simulink model "Testing_User_defined_Function"  (R2019b)
settings: Solver=VariableStepAuto  StartTime=0.0  StopTime=10  FixedStep=0.0001  RelTol=1e-3
values from neighbouring files (symbols this model uses):
  B = (NL_current*Km)/NL_speed    (= 7.06678023853e-07)    [DCX19_Motor_Calculations.m]
  J = 2.72*10^-7    (= 2.72e-07)    [DCX19_Motor_Calculations.m]
  Kb = 1/(268*(2*pi/60))    (= 0.0356317036773)    [DCX19_Motor_Calculations.m]
  Kd = (K - Kp)/filter_pole    [DCX19_Motor_Calculations.m]
  Ki = ((z1*z2)*K)/filter_pole    [DCX19_Motor_Calculations.m]
  Km = 35.6*10^-3    (= 0.0356)    [DCX19_Motor_Calculations.m]
  Kp = (K*(z1 + z2) - Ki)/filter_pole    [DCX19_Motor_Calculations.m]
  L = 1.320*10^-3    (= 0.00132)    [DCX19_Motor_Calculations.m]
  res = (2*pi)/CPR    (= 0.0490873852123)    [DCX19_Motor_Calculations.m]
undefined symbols (not defined in the file or in its folder): R
libraries: cstblocks x2, simulink x1
settings Model: Creator=harsh  LastModifiedBy=harsh

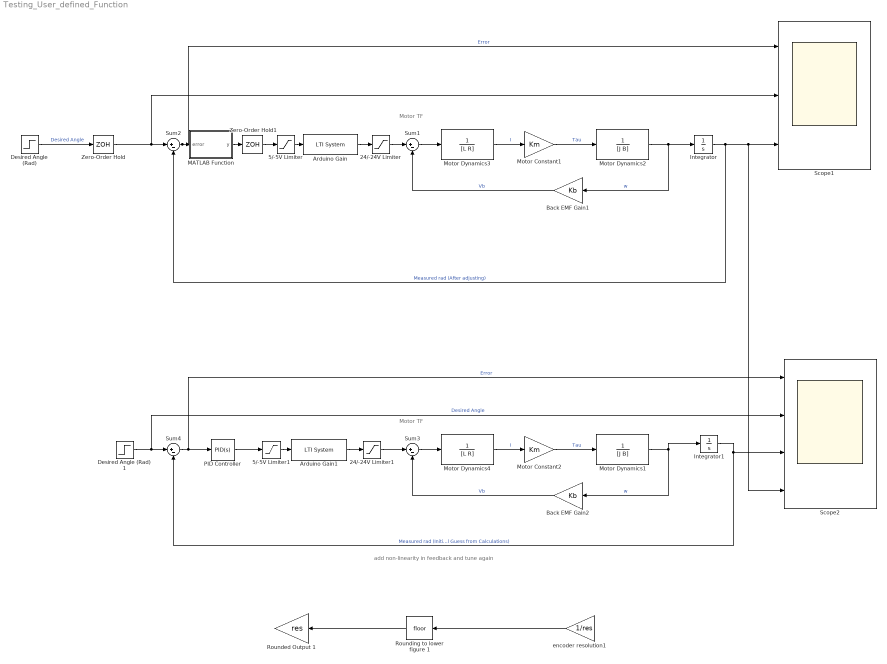
== system Testing_User_defined_Function ==
  note: add non-linearity in feedback and tune again
  note: Motor TF
  note: Motor TF
  24/-24V Limiter : Saturate  UpperLimit=5  LowerLimit=-5
  24/-24V Limiter1 : Saturate  UpperLimit=5  LowerLimit=-5
  5/-5V Limiter : Saturate  UpperLimit=5  LowerLimit=-5
  5/-5V Limiter1 : Saturate  UpperLimit=5  LowerLimit=-5
  Arduino Gain : cstblocks/LTI System  sys=OPAMP  IC=[]
  Arduino Gain1 : cstblocks/LTI System  sys=OPAMP  IC=[]
  Back EMF Gain1 : Gain  Gain=Kb
  Back EMF Gain2 : Gain  Gain=Kb
  "Desired Angle (Rad) " : Step  After=1.5707  SampleTime=0
  Desired Angle (Rad) 1 : Step  After=1.5707  SampleTime=0
  Integrator : Integrator
  Integrator1 : Integrator
  MATLAB Function : MATLAB Function  TreatAsAtomicUnit=on
  Motor Constant1 : Gain  Gain=Km
  Motor Constant2 : Gain  Gain=Km
  Motor Dynamics1 : TransferFcn  Denominator=[J B]
  Motor Dynamics2 : TransferFcn  Denominator=[J B]
  Motor Dynamics3 : TransferFcn  Denominator=[L R]
  Motor Dynamics4 : TransferFcn  Denominator=[L R]
  PID Controller : simulink/Continuous/PID Controller  Controller=PID  Form=Parallel  TimeDomain=Continuous-time  SampleTime=-1  IntegratorMethod=Forward Euler  FilterMethod=Forward Euler  ControllerParametersSource=internal  P=Kp  I=Ki  D=Kd  UseFilter=on  N=5000  TunerSelectOption=Transfer Function Based (PID Tuner App)  InitialConditionSource=internal  InitialConditionForIntegrator=0  InitialConditionForFilter=0  DifferentiatorICPrevScaledInput=0  ExternalReset=none  TrackingMode=off  Kt=1  LimitOutput=off  UpperSaturationLimit=inf  LowerSaturationLimit=-inf  LinearizeAsGain=on  AntiWindupMode=none  Kb=1  POutMin=[]  POutMax=[]  IOutMin=[]  IOutMax=[]  DOutMin=[]  DOutMax=[]  NOutMin=[]  NOutMax=[]  SumOutMin=[]  SumOutMax=[]  SaturationOutMin=[]  SaturationOutMax=[]  PParamMin=[]  PParamMax=[]  IParamMin=[]  IParamMax=[]  DParamMin=[]  DParamMax=[]  NParamMin=[]  NParamMax=[]  KbParamMin=[]  KbParamMax=[]  KtParamMin=[]  KtParamMax=[]  KbOutMin=[]  KbOutMax=[]  KtOutMin=[]  KtOutMax=[]  IntegratorOutMin=[]  IntegratorOutMax=[]  FilterOutMin=[]  FilterOutMax=[]  SumI1OutMin=[]  SumI1OutMax=[]  SumI2OutMin=[]  SumI2OutMax=[]  SumI3OutMin=[]  SumI3OutMax=[]  SumI4OutMin=[]  SumI4OutMax=[]  SumDOutMin=[]  SumDOutMax=[]  DifferentiatorOutMin=[]  DifferentiatorOutMax=[]  FilterDiffOutCoefMin=[]  FilterDiffOutCoefMax=[]  ReciprocalOutMin=[]  ReciprocalOutMax=[]  SumDenOutMin=[]  SumDenOutMax=[]  SumNumOutMin=[]  SumNumOutMax=[]  DivideOutMin=[]  DivideOutMax=[]  IntegratorContinuousStateAttributes=''  IntegratorStateMustResolveToSignalObject=off  IntegratorRTWStateStorageClass=Auto  FilterContinuousStateAttributes=''  FilterStateMustResolveToSignalObject=off  FilterRTWStateStorageClass=Auto  ParallelPVariant=InternalParameters  IdealPVariant=Disabled  IVariant=InternalParameters  DVariant=InternalParameters  IntegratorVariant=Continuous  SatVariant=Disabled  AWVariant=Passthrough  PCopyVariant=Disabled  TRVariant=Disabled  FdbkBlocksVariant=Forward  IdealPFdbkVariant=Disabled  SatFdbkVariant=Disabled  DerivativeFilterVariant=ContFilter  NVariant=InternalParameters  NCopyVariant=Disabled  FilterICVariant=InternalICsFilter  IntegratorICVariant=InternalICs  ExternalResetVariant=Disabled  TRSumVariant=Passthrough  SumFdbkVariant=Disabled  SumVariant=Sum_PID
  Rounded Output 1 : Gain  Gain=res
  Rounding to lower figure 1 : Rounding
  Scope1 : Scope  NumInputPorts=3
  Scope2 : Scope  NumInputPorts=4
  Sum{1..4} (4 alike) : Sum  Inputs=|+-
  Zero-Order Hold : ZeroOrderHold  SampleTime=0.0001
  Zero-Order Hold1 : ZeroOrderHold  SampleTime=0.0001
  encoder resolution1 : Gain  Gain=1/res
  wires:
  5/-5V Limiter/1 -> Arduino Gain/1
  Sum1/1 -> Motor Dynamics3/1
  Arduino Gain/1 -> 24/-24V Limiter/1
  Back EMF Gain1/1 -> Sum1/2  "Vb"
  Motor Dynamics3/1 -> Motor Constant1/1  "I"
  24/-24V Limiter/1 -> Sum1/1
  Motor Constant1/1 -> Motor Dynamics2/1  "Tau"
  "Desired Angle (Rad) "/1 -> Zero-Order Hold/1  "Desired Angle"
  Sum2/1 -> Scope1/1, MATLAB Function/1(error)  "Error"
  Motor Dynamics2/1 -> Integrator/1, Back EMF Gain1/1  "w"
  Motor Dynamics1/1 -> Back EMF Gain2/1, Integrator1/1  "w"
  Desired Angle (Rad) 1/1 -> Scope2/2, Sum4/1  "Desired Angle"
  PID Controller/1 -> 5/-5V Limiter1/1
  Sum4/1 -> PID Controller/1, Scope2/1  "Error"
  Motor Dynamics4/1 -> Motor Constant2/1  "I"
  Motor Constant2/1 -> Motor Dynamics1/1  "Tau"
  24/-24V Limiter1/1 -> Sum3/1
  Arduino Gain1/1 -> 24/-24V Limiter1/1
  Back EMF Gain2/1 -> Sum3/2  "Vb"
  5/-5V Limiter1/1 -> Arduino Gain1/1
  Sum3/1 -> Motor Dynamics4/1
  Integrator/1 -> Scope2/4, Scope1/3, Sum2/2  "Measured rad (After adjusting)"
  Integrator1/1 -> Sum4/2, Scope2/3  "Measured rad (Initial Guess from Calculations)"
  encoder resolution1/1 -> Rounding to lower figure 1/1
  Rounding to lower figure 1/1 -> Rounded Output 1/1
  Zero-Order Hold/1 -> Scope1/2, Sum2/1
  MATLAB Function/1(y) -> Zero-Order Hold1/1
  Zero-Order Hold1/1 -> 5/-5V Limiter/1

== matlab function Testing_User_defined_Function/MATLAB Function ==
  settings: updateMethod=DISCRETE
  data: error input; y output
function y = fcn(error)

persistent previous_error;                  %previous error = current error for next iteration, initially set to 0;
persistent Ki_output;                        %need as persistent variable for Ki_output = Ki_output + (...)
persistent ept;                             %constant vector of exponentials (p*e^(-p*n*Ts)) where n = 1.....#of samples we want to average
persistent unweighted_differential_outputs;  %vector used for dot product with ept, shifted at each cycle. 

if isempty(previous_error)
    previous_error = 0;
end

%Trial values for testing against Built in PID block
Kp = 0.223809;
Ki = 0.011836;
Kd = 0.012272;

Ts = 0.0001;    %Controller frequency from Arduino assumed to be 10kHz.

%--------P controller part------------------
Kp_output = Kp*error;    

%---------I controller part-----------------

%Initializing Ki_output
if isempty(Ki_output)
    Ki_output = 0;
end

Ki_output = Ki_output + Ki*[(error + previous_error)/2]*Ts; %cumulative areas of trapeziums

%----------D controller part----------------
controlfreq = 10000; %Hz
filter_pole = 4000;  %big pole because we don't care much about averaging but we do care a lot about delay. (signal is not noisy)
n = 4*controlfreq/filter_pole;  %We are averaging 80 samples in this example


%Now, we initialize the ept vector (will remain constant valued throughout the program)
if isempty(ept)
    ept = zeros(1,n);
    for i = 1:n
        ept(i) = filter_pole*1.132*exp(-filter_pole*i*Ts);
    end
    %We want Ts*sum(ept) = 1 but this is not the case normally, so we have to scale the ept such that we get a sum
    %of 1. To account for discretization error, we scale it by multiplying it by 1.132 in this example. 
end

if isempty(unweighted_differential_outputs)
    unweighted_differential_outputs = zeros(1,n);
end 

unweighted_differential_outputs(1) = (error - previous_error); 
filtered_derivative = dot(ept,unweighted_differential_outputs);

Kd_output = Kd*filtered_derivative;

n2 = n+1; %n2 = 9
for count = 1:(n-1) %1:7 in this example
    unweighted_differential_outputs(n2-count) = unweighted_differential_outputs(n2 - count - 1);    %shift values by one index, and in next loop calculate one more new slope at index 1 (starting index)
end 

y = Kp_output + Ki_output + Kd_output;

previous_error = error; %this will help us move on to get new values for Ki and Kd

end
